simulink model "dem_uDAQ_simulink"  (R2020b)
settings: Solver=VariableStepAuto  StartTime=0.0  StopTime=10  RelTol=1e-3
values from neighbouring files (symbols this model uses):
  simparams =     [uDAQ28LT_variables.mat]    (also in uDAQ_variables.m = struct)
libraries: uDAQ28LT_lib x2
settings Model: Creator=dp  LastModifiedBy=udaq

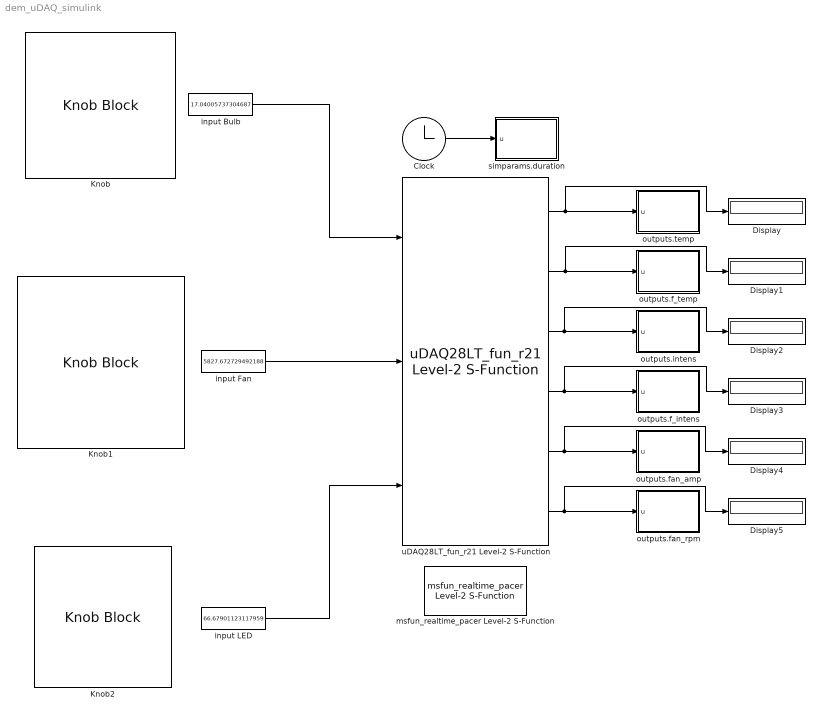
== system dem_uDAQ_simulink ==
  Clock : Clock
  Display{,1..5} (6 alike) : Display
  Knob : KnobBlock  ScaleMax=20
  Knob1 : KnobBlock  ScaleMax=6000
  Knob2 : KnobBlock
  input Bulb : Constant  Value=17.04005737304687  SampleTime=simparams.Ts
  input Fan : Constant  Value=5827.672729492188  SampleTime=simparams.Ts
  input LED : Constant  Value=66.67901123117959  SampleTime=simparams.Ts
  msfun_realtime_pacer Level-2 S-Function : uDAQ28LT_lib/msfun_realtime_pacer Level-2 S-Function  simTimePerRealTime=1
  outputs.f_intens : MATLAB Function  TreatAsAtomicUnit=on  SystemSampleTime=simparams.Ts
  outputs.f_temp : MATLAB Function  TreatAsAtomicUnit=on  SystemSampleTime=simparams.Ts
  outputs.fan_amp : MATLAB Function  TreatAsAtomicUnit=on  SystemSampleTime=simparams.Ts
  outputs.fan_rpm : MATLAB Function  TreatAsAtomicUnit=on  SystemSampleTime=simparams.Ts
  outputs.intens : MATLAB Function  TreatAsAtomicUnit=on  SystemSampleTime=simparams.Ts
  outputs.temp : MATLAB Function  TreatAsAtomicUnit=on  SystemSampleTime=simparams.Ts
  simparams.duration : MATLAB Function  TreatAsAtomicUnit=on  SystemSampleTime=simparams.Ts
  uDAQ28LT_fun_r21 Level-2 S-Function : uDAQ28LT_lib/uDAQ28LT_fun_r21 Level-2 S-Function  com='/dev/ttyUSB0,dem_uDAQ_output.txt'  baud=256000  Ts=0.1
  wires:
  uDAQ28LT_fun_r21 Level-2 S-Function/6 -> outputs.fan_rpm/1(u), Display5/1
  uDAQ28LT_fun_r21 Level-2 S-Function/5 -> outputs.fan_amp/1(u), Display4/1
  uDAQ28LT_fun_r21 Level-2 S-Function/4 -> outputs.f_intens/1(u), Display3/1
  uDAQ28LT_fun_r21 Level-2 S-Function/3 -> outputs.intens/1(u), Display2/1
  uDAQ28LT_fun_r21 Level-2 S-Function/1 -> outputs.temp/1(u), Display/1
  uDAQ28LT_fun_r21 Level-2 S-Function/2 -> outputs.f_temp/1(u), Display1/1
  Clock/1 -> simparams.duration/1(u)
  input Fan/1 -> uDAQ28LT_fun_r21 Level-2 S-Function/2
  input LED/1 -> uDAQ28LT_fun_r21 Level-2 S-Function/3
  input Bulb/1 -> uDAQ28LT_fun_r21 Level-2 S-Function/1

== matlab function dem_uDAQ_simulink/simparams.duration ==
  data: u input
function fcn(u)
coder.extrinsic('evalin');
evalin('base',sprintf('simparams.duration(end+1)=%f;',u));
end

== matlab function dem_uDAQ_simulink/outputs.temp ==
  data: u input
function fcn(u)
coder.extrinsic('evalin');
evalin('base',sprintf('outputs.temp(end+1)=%f;',u));
end

== matlab function dem_uDAQ_simulink/outputs.intens ==
  data: u input
function fcn(u)
coder.extrinsic('evalin');
evalin('base',sprintf('outputs.intens(end+1)=%f;',u));
end

== matlab function dem_uDAQ_simulink/outputs.f_intens ==
  data: u input
function fcn(u)
coder.extrinsic('evalin');
evalin('base',sprintf('outputs.f_intens(end+1)=%f;',u));
end

== matlab function dem_uDAQ_simulink/outputs.fan_amp ==
  data: u input
function fcn(u)
coder.extrinsic('evalin');
evalin('base',sprintf('outputs.fan_amp(end+1)=%f;',u));
end

== matlab function dem_uDAQ_simulink/outputs.fan_rpm ==
  data: u input
function fcn(u)
coder.extrinsic('evalin');
evalin('base',sprintf('outputs.fan_rpm(end+1)=%f;',u));
end

== matlab function dem_uDAQ_simulink/outputs.f_temp ==
  data: u input
function fcn(u)
coder.extrinsic('evalin');
evalin('base',sprintf('outputs.f_temp(end+1)=%f;',u));
end
